simulink model "Control_PID"  (Simulink 7.5)
settings: Solver=ode45  StartTime=0.0  StopTime=1.0  RelTol=1e-3
settings Model: Creator=davito  LastModifiedBy=davito

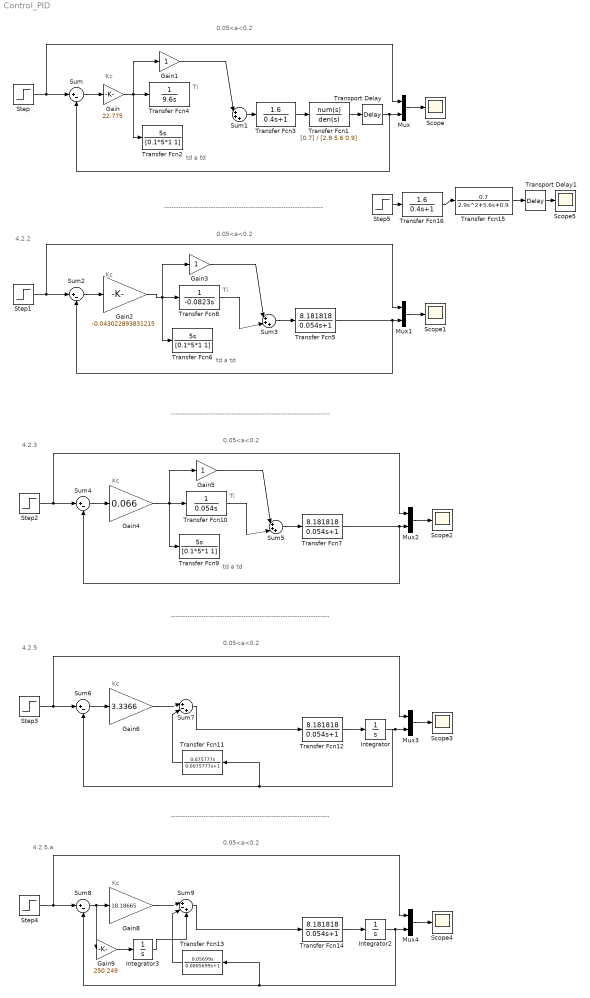
== system Control_PID ==
  note: Kc
  note: Ti
  note: td
      | a td
  note: 0.05<a<0.2
  note: Kc
  note: Ti
  note: td
      | a td
  note: 0.05<a<0.2
  note: 4.2.2
  note: --------------------------------------------------------------------
  note: Kc
  note: Ti
  note: td
      | a td
  note: 0.05<a<0.2
  note: 4.2.3
  note: --------------------------------------------------------------------
  note: Kc
  note: 0.05<a<0.2
  note: 4.2.5
  note: --------------------------------------------------------------------
  note: Kc
  note: 0.05<a<0.2
  note: 4.2.5.a
  note: --------------------------------------------------------------------
  Gain : Gain  Gain=22.775  ParameterDataType=fixdt(1, 16)  ParameterScaling=2^0  OutDataType=fixdt(1, 16)  OutScaling=2^0
  Gain1 : Gain  ParameterDataType=fixdt(1, 16)  ParameterScaling=2^0  OutDataType=fixdt(1, 16)  OutScaling=2^0
  Gain2 : Gain  Gain=-0.043022893831215  ParameterDataType=fixdt(1, 16)  ParameterScaling=2^0  OutDataType=fixdt(1, 16)  OutScaling=2^0
  Gain3 : Gain  ParameterDataType=fixdt(1, 16)  ParameterScaling=2^0  OutDataType=fixdt(1, 16)  OutScaling=2^0
  Gain4 : Gain  Gain=0.066  ParameterDataType=fixdt(1, 16)  ParameterScaling=2^0  OutDataType=fixdt(1, 16)  OutScaling=2^0
  Gain5 : Gain  ParameterDataType=fixdt(1, 16)  ParameterScaling=2^0  OutDataType=fixdt(1, 16)  OutScaling=2^0
  Gain6 : Gain  Gain=3.3366  ParameterDataType=fixdt(1, 16)  ParameterScaling=2^0  OutDataType=fixdt(1, 16)  OutScaling=2^0
  Gain8 : Gain  Gain=18.18665  ParameterDataType=fixdt(1, 16)  ParameterScaling=2^0  OutDataType=fixdt(1, 16)  OutScaling=2^0
  Gain9 : Gain  Gain=250.249  ParameterDataType=fixdt(1, 16)  ParameterScaling=2^0  OutDataType=fixdt(1, 16)  OutScaling=2^0
  Integrator : Integrator
  Integrator2 : Integrator
  Integrator3 : Integrator
  Mux{,1..4} (5 alike) : Mux  Inputs=2
  Scope{,1..5} (6 alike) : Scope
      Scope settings: YMin=0  YMax=30
      Scope1 settings: YMin=100  YMax=100
      Scope2 settings: YMin=0  YMax=1  SaveName=ScopeData2
      Scope3 settings: YMin=0  YMax=1  SaveName=ScopeData3
      Scope4 settings: YMin=0  YMax=1  SaveName=ScopeData4
      Scope5 settings: YMin=0  YMax=30  SaveName=ScopeData5
  Step : Step  Time=0  SampleTime=0
  Step{1..4} (4 alike) : Step  Time=0  After=100  SampleTime=0
  Step5 : Step  Time=0  SampleTime=0
  Sum{,2,4,6,8} (5 alike) : Sum  Inputs=|+-  OutDataType=fixdt(1, 16)  OutScaling=2^0
  Sum1 : Sum  Inputs=|+++  OutDataType=fixdt(1, 16)  OutScaling=2^0
  Sum3 : Sum  Inputs=|+++  OutDataType=fixdt(1, 16)  OutScaling=2^0
  Sum5 : Sum  Inputs=|+++  OutDataType=fixdt(1, 16)  OutScaling=2^0
  Sum7 : Sum  Inputs=|+-+  OutDataType=fixdt(1, 16)  OutScaling=2^0
  Sum9 : Sum  Inputs=|+-+  OutDataType=fixdt(1, 16)  OutScaling=2^0
  Transfer Fcn1 : TransferFcn  Numerator=[0.7]  Denominator=[2.9 5.6 0.9]
  Transfer Fcn10 : TransferFcn  Denominator=[0.054 0]
  Transfer Fcn11 : TransferFcn  Numerator=[0.075777 0]  Denominator=[0.0075777 1]
  Transfer Fcn{5,7,12,14} (4 alike) : TransferFcn  Numerator=[8.181818]  Denominator=[0.054 1]
  Transfer Fcn13 : TransferFcn  Numerator=[0.05699 0]  Denominator=[0.0005699 1]
  Transfer Fcn15 : TransferFcn  Numerator=[0.7]  Denominator=[2.9 5.6 0.9]
  Transfer Fcn16 : TransferFcn  Numerator=[1.6]  Denominator=[0.4 1]
  Transfer Fcn2 : TransferFcn  Numerator=[5 0]  Denominator=[0.1*5*1 1]
  Transfer Fcn3 : TransferFcn  Numerator=[1.6]  Denominator=[0.4 1]
  Transfer Fcn4 : TransferFcn  Denominator=[9.6 0]
  Transfer Fcn6 : TransferFcn  Numerator=[5 0]  Denominator=[0.1*5*1 1]
  Transfer Fcn8 : TransferFcn  Denominator=[-0.0823 0]
  Transfer Fcn9 : TransferFcn  Numerator=[5 0]  Denominator=[0.1*5*1 1]
  Transport Delay : TransportDelay  DelayTime=2
  Transport Delay1 : TransportDelay  DelayTime=2
  wires:
  Step/1 -> Sum/1, Mux/1
  Transfer Fcn3/1 -> Transfer Fcn1/1
  Sum1/1 -> Transfer Fcn3/1
  Gain1/1 -> Sum1/1
  Gain/1 -> Transfer Fcn4/1, Transfer Fcn2/1, Gain1/1
  Sum/1 -> Gain/1
  Mux/1 -> Scope/1
  Step1/1 -> Mux1/1, Sum2/1
  Transfer Fcn5/1 -> Sum2/2, Mux1/2
  Sum3/1 -> Transfer Fcn5/1
  Gain3/1 -> Sum3/1
  Gain2/1 -> Gain3/1, Transfer Fcn6/1, Transfer Fcn8/1
  Sum2/1 -> Gain2/1
  Mux1/1 -> Scope1/1
  Transfer Fcn8/1 -> Sum3/2
  Step2/1 -> Sum4/1, Mux2/1
  Transfer Fcn7/1 -> Mux2/2, Sum4/2
  Sum5/1 -> Transfer Fcn7/1
  Gain5/1 -> Sum5/1
  Gain4/1 -> Transfer Fcn10/1, Transfer Fcn9/1, Gain5/1
  Sum4/1 -> Gain4/1
  Mux2/1 -> Scope2/1
  Transfer Fcn10/1 -> Sum5/2
  Step3/1 -> Mux3/1, Sum6/1
  Sum7/1 -> Transfer Fcn12/1
  Sum6/1 -> Gain6/1
  Mux3/1 -> Scope3/1
  Transfer Fcn12/1 -> Integrator/1
  Integrator/1 -> Mux3/2, Transfer Fcn11/1, Sum6/2
  Gain6/1 -> Sum7/1
  Transfer Fcn11/1 -> Sum7/2
  Step4/1 -> Sum8/1, Mux4/1
  Sum9/1 -> Transfer Fcn14/1
  Sum8/1 -> Gain9/1, Gain8/1
  Mux4/1 -> Scope4/1
  Transfer Fcn14/1 -> Integrator2/1
  Integrator2/1 -> Sum8/2, Transfer Fcn13/1, Mux4/2
  Gain8/1 -> Sum9/1
  Transfer Fcn13/1 -> Sum9/2
  Gain9/1 -> Integrator3/1
  Integrator3/1 -> Sum9/3
  Transfer Fcn1/1 -> Transport Delay/1
  Transport Delay/1 -> Mux/2, Sum/2
  Transfer Fcn16/1 -> Transfer Fcn15/1
  Transfer Fcn15/1 -> Transport Delay1/1
  Step5/1 -> Transfer Fcn16/1
  Transport Delay1/1 -> Scope5/1
